simulink model "a4_smlk"  (R2023b)
settings: Solver=VariableStepAuto  StartTime=0.0  StopTime=50  FixedStep=.02  RelTol=1e-3
libraries: simulink x1
settings Model: Creator=LUCAS  LastModifiedBy=LUCAS

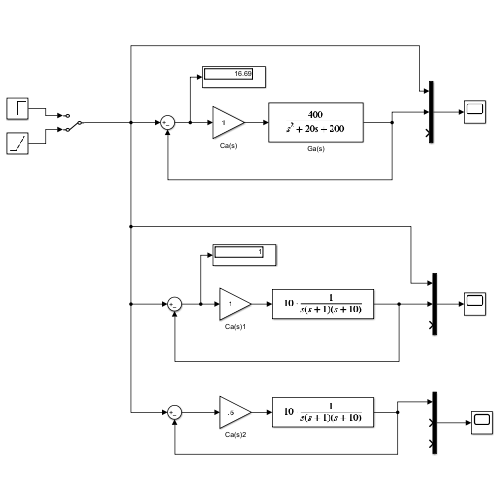
[thumbnail: Simulink's stored preview of the top-level diagram]
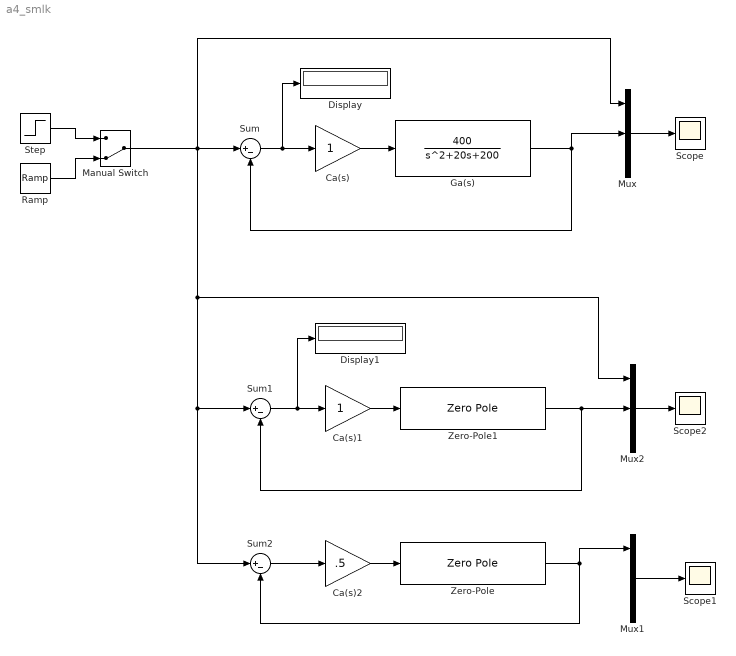
== system a4_smlk ==
  Ca(s) : Gain
  Ca(s)1 : Gain
  Ca(s)2 : Gain  Gain=.5
  Display : Display
  Display1 : Display
  Ga(s) : TransferFcn  Numerator=[400]  Denominator=[1 20 200]
  Manual Switch : ManualSwitch  CurrentSetting=0
  Mux : Mux  Inputs=3
  Mux1 : Mux  Inputs=3
  Mux2 : Mux  Inputs=3
  Ramp : simulink/Sources/Ramp  slope=1  start=0  InitialOutput=0
  Scope : Scope
  Scope1 : Scope
  Scope2 : Scope
  Step : Step  SampleTime=0
  Sum : Sum  Inputs=|+-
  Sum1 : Sum  Inputs=|+-
  Sum2 : Sum  Inputs=|+-
  Zero-Pole : ZeroPole  Zeros=[]  Poles=[0 -1 -10]  Gain=10
  Zero-Pole1 : ZeroPole  Zeros=[]  Poles=[0 -1 -10]  Gain=10
  wires:
  Ca(s)/1 -> Ga(s)/1
  Ga(s)/1 -> Mux/2, Sum/2
  Sum/1 -> Display/1, Ca(s)/1
  Ca(s)1/1 -> Zero-Pole1/1
  Mux/1 -> Scope/1
  Sum2/1 -> Ca(s)2/1
  Ca(s)2/1 -> Zero-Pole/1
  Zero-Pole/1 -> Mux1/1, Sum2/2
  Mux1/1 -> Scope1/1
  Manual Switch/1 -> Mux/1, Sum2/1, Sum1/1, Mux2/1, Sum/1
  Ramp/1 -> Manual Switch/2
  Step/1 -> Manual Switch/1
  Mux2/1 -> Scope2/1
  Zero-Pole1/1 -> Mux2/2, Sum1/2
  Sum1/1 -> Display1/1, Ca(s)1/1
